simulink model "bilinear_transf"  (R2020a)
settings: Solver=VariableStepAuto  StartTime=0.0  StopTime=10.0  RelTol=1e-3
libraries: dspsrcs4 x1
settings Model: Creator=kolep  LastModifiedBy=kolep

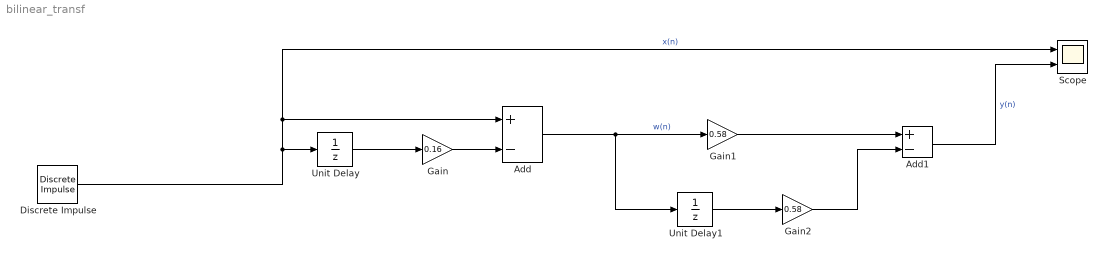
== system bilinear_transf ==
  Add : Sum  Inputs=+-
  Add1 : Sum  Inputs=+-
  Discrete Impulse : dspsrcs4/Discrete  Impulse  Delay=0  SampleTime=1  FrameSample=1  OutputFrames=off  dataType=double  isSigned=on  wordLen=16  udDataType=sfix(16)  fracBitsMode=Best precision  numFracBits=15  OutDataTypeStr=double  LastOutDataTypeStr=double
  Gain : Gain  Gain=0.16
  Gain1 : Gain  Gain=0.58
  Gain2 : Gain  Gain=0.58
  Scope : Scope  NumInputPorts=2
  Unit Delay : UnitDelay  SampleTime=-1  HasFrameUpgradeWarning=on
  Unit Delay1 : UnitDelay  SampleTime=-1  HasFrameUpgradeWarning=on
  wires:
  Gain1/1 -> Add1/1
  Unit Delay/1 -> Gain/1
  Add/1 -> Unit Delay1/1, Gain1/1  "w(n)"
  Unit Delay1/1 -> Gain2/1
  Gain/1 -> Add/2
  Discrete Impulse/1 -> Scope/1, Add/1, Unit Delay/1  "x(n)"
  Gain2/1 -> Add1/2
  Add1/1 -> Scope/2  "y(n)"
